simulink model "transmitFMTone_USRP"  (R2017a)
settings: Solver=VariableStepAuto  StartTime=0.0  StopTime=inf  RelTol=1e-3
libraries: commanabbnd3 x1, commrflib2 x1, commsdrhw_v2 x1, dspsrcs4 x1
settings Model: Creator=prust  LastModifiedBy=prust

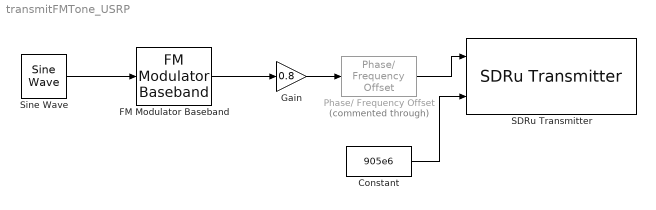
== system transmitFMTone_USRP ==
  Constant : Constant  Value=905e6
  FM Modulator Baseband : commanabbnd3/FM Modulator Baseband  FrequencyDeviation=2e3  SimulateUsing=Code generation
      settings: SourceProductName=Communications System Toolbox  SourceProductBaseCode=CM
  Gain : Gain  Gain=0.8
  Phase/ Frequency Offset : commrflib2/Phase// Frequency Offset  Commented=through  phaseOffset=0  freqPort=off  freqOffset=50e3
      settings: SourceProductName=Communications System Toolbox
  SDRu Transmitter : commsdrhw_v2/SDRu Transmitter  SourceLibraryInfo="This block requires <a href=\"http://www.mathworks.com/hardware-support/usrp.html\">Communications System Toolbox Support Package for USRP Radio</a>"  rxtx=tx  platform=B200  USRP2_IP='192.168.10.2'  USRP_IP_X300='192.168.10.2'  USRP_IP_X310='192.168.10.2'  USRP_serialNumB200='30703A1'  USRP_serialNumB210=''  ChannelMapping=1  centerFrequency=905e6  centerFrequencySrc=Input port  loOffset=0  loOffsetSrc=Dialog  PPSSource=Internal  clockSource=Internal  masterClkRateB200=32e6  masterClkRateB210=32e6  masterClkRateX300=200e6  masterClkRateX310=200e6  masterClkRateParam=32000000  gain=45  gainSrc=Dialog  decimInterp=512  decimInterpSrc=Dialog  TransportDataType=int16  USRP2_IP_NUM=[51 48 55 48 51 65 49]  frameLength=362  outputDatatype=Same as transport data type  overrunUnderrunPort=off  sampleTime=1  dboardInfo=|  HOST_DATA_PORT=30000  HOST_CONTROL_PORT=30001  USRP2_DATA_PORT=32769  USRP2_CONTROL_PORT=32768  bufferMode=Continuous streaming  EnableBurstMode=off  NumFramesInBurst=100  USRP_ID='30703A1'
      | dbid: 0
      |           dbName: 'no db found'
      |          freqMin: 0
      |          freqMax: 0
      |          gainMin: 0
      |          gainMax: 0
      |     gainStepSize: 0
      settings: SourceProductName=Communications System Toolbox Support Package for USRP(R) Radio  SourceProductBaseCode=USRP
  Sine Wave : dspsrcs4/Sine Wave  Amplitude=1  Frequency=2100  Phase=0  SampleMode=Discrete  OutComplex=Real  CompMethod=Trigonometric fcn  TableSize=Speed  SampleTime=1/62500  SamplesPerFrame=10000  ResetState=Restart at time zero  OutputFrames=off  dataType=double  wordLen=16  udDataType=sfix(16)  fracBitsMode=Best precision  numFracBits=15  OutDataTypeStr=double  LastOutDataTypeStr=double
  wires:
  Sine Wave/1 -> FM Modulator Baseband/1
  FM Modulator Baseband/1 -> Gain/1
  Constant/1 -> SDRu Transmitter/2
  Gain/1 -> Phase/ Frequency Offset/1
  Phase/ Frequency Offset/1 -> SDRu Transmitter/1
